simulink subsystem "LO"  (R2024a)
settings: Solver=VariableStepAuto  StartTime=0.0  StopTime=10.0  RelTol=1e-3
undefined symbols (not defined in the file): A, B, C, D, L_LO
libraries: observer x1
settings Model: Creator=Bocchio  LastModifiedBy=Bocchio

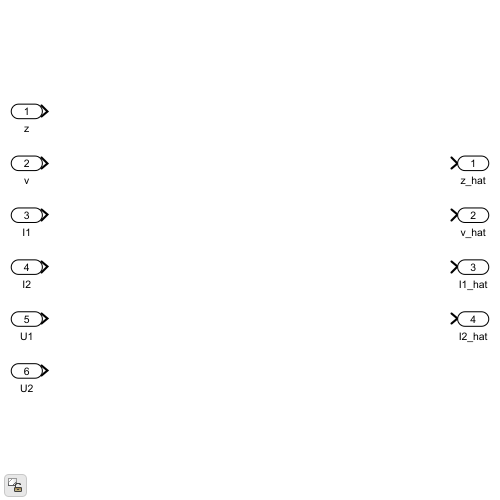
[thumbnail: Simulink's stored preview of the top-level diagram]
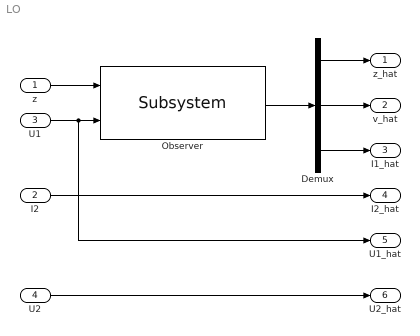
== system LO ==
  z : Inport
  I2 : Inport  Port=2
  U1 : Inport  Port=3
  U2 : Inport  Port=4
  Demux : Demux  Outputs=3
  Observer : observer/Subsystem  L=L_LO  A=A  B=B  C=C  D=D
  z_hat : Outport
  v_hat : Outport  Port=2
  I1_hat : Outport  Port=3
  I2_hat : Outport  Port=4
  U1_hat : Outport  Port=5
  U2_hat : Outport  Port=6
  wires:
  Demux/1 -> z_hat/1
  Demux/2 -> v_hat/1
  Demux/3 -> I1_hat/1
  I2/1 -> I2_hat/1
  Observer/1 -> Demux/1
  U1/1 -> Observer/2, U1_hat/1
  z/1 -> Observer/1
  U2/1 -> U2_hat/1
